simulink model "car_suspension"  (R2023a)
settings: Solver=VariableStepAuto  StartTime=0.0  StopTime=1000  RelTol=1e-3
values from neighbouring files (symbols this model uses):
  x_road = [0 0.101711 0.203422 0.305133 0.406844 0.508555 0.610266 0.711977 0.813688 0.915399 1.01711 1.118821 ... (27038 elements, 27038x1)]    [road_profile.mat]
  z_road = [-0.000630002 -8.000197e-05 0.000269998 0.000749998 0.001499998 0.002299998 0.003329998 0.004419998 0.005089998 0.005469998 0.005659998 0.005699998 ... (27038 elements, 27038x1)]    [road_profile.mat]
undefined symbols (not defined in the file or in its folder): A, B, C, D, den, init_c, num, vel, x_start, x_stop
libraries: simulink x2
settings Model: Creator=m260477  LastModifiedBy=m260477

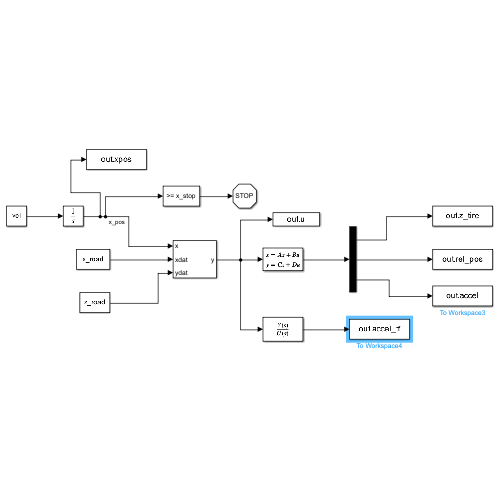
[thumbnail: Simulink's stored preview of the top-level diagram]
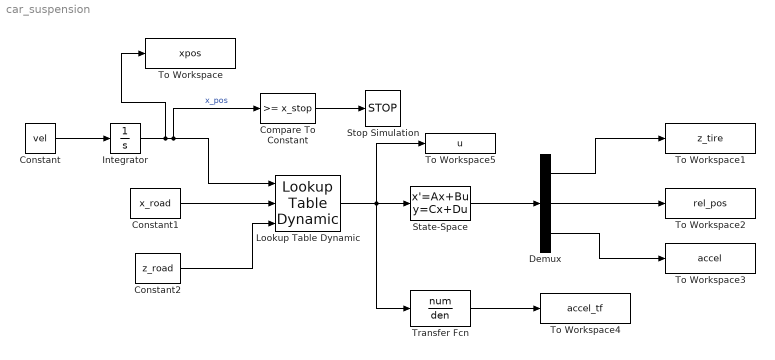
== system car_suspension ==
  Compare To Constant : simulink/Logic and Bit Operations/Compare To Constant  relop=>=  const=x_stop  OutDataTypeStr=boolean
  Constant : Constant  Value=vel
  Constant1 : Constant  Value=x_road
  Constant2 : Constant  Value=z_road
  Demux : Demux  Outputs=3
  Integrator : Integrator  InitialCondition=x_start
  Lookup Table Dynamic : simulink/Lookup Tables/Lookup Table Dynamic  LookUpMeth=Interpolation-Use End Values  OutDataType=fixdt('double')  OutScaling=2^-10  OutputDataTypeScalingMode=Specify via dialog  OutDataTypeStr=double  DoSatur=off
  State-Space : StateSpace  A=A  B=B  C=C  D=D  InitialCondition=init_c
  Stop Simulation : Stop
  To Workspace : ToWorkspace  VariableName=xpos  SaveFormat=Timeseries  SampleTime=-1
  To Workspace1 : ToWorkspace  VariableName=z_tire  SaveFormat=Timeseries  SampleTime=-1
  To Workspace2 : ToWorkspace  VariableName=rel_pos  SaveFormat=Timeseries  SampleTime=-1
  To Workspace3 : ToWorkspace  VariableName=accel  SaveFormat=Timeseries  SampleTime=-1
  To Workspace4 : ToWorkspace  VariableName=accel_tf  SaveFormat=Timeseries  SampleTime=-1
  To Workspace5 : ToWorkspace  VariableName=u  SaveFormat=Timeseries  SampleTime=-1
  Transfer Fcn : TransferFcn  Numerator=num  Denominator=den
  wires:
  Integrator/1 -> To Workspace/1, Compare To Constant/1, Lookup Table Dynamic/1  "x_pos"
  Demux/2 -> To Workspace2/1
  Demux/1 -> To Workspace1/1
  Demux/3 -> To Workspace3/1
  State-Space/1 -> Demux/1
  Lookup Table Dynamic/1 -> Transfer Fcn/1, To Workspace5/1, State-Space/1
  Constant1/1 -> Lookup Table Dynamic/2
  Constant2/1 -> Lookup Table Dynamic/3
  Compare To Constant/1 -> Stop Simulation/1
  Constant/1 -> Integrator/1
  Transfer Fcn/1 -> To Workspace4/1
